simulink model "MODEL_SS_withSCC_Emily"  (R2024b)
settings: Solver=VariableStepAuto  StartTime=0.0  StopTime=40  RelTol=1e-3
PostLoadFcn:
  | Cconst = 0.15915494327;
  | Kp = [76; 141.7; 139.6; 114.2]*Cconst/60;
  | Tp = [14.4; 19.1; 9.39; 9.12];
  | Tg = 0.38*ones(4,1);
  | R = 3/60*ones(4,1);
  | Bagc = [0.416; 0.377; 0.378; 0.388]*60;
  | Kagc = [0.75; 0.25; 0.5; 0.5]*(-0.131);
  | Kdc = ones(4,1);
  | 
  | T = zeros(4,4);
  | T(1, 2) = 0.029;
  | T(1, 3) = 0.0143;
  | T(1, 4) = 0.0099;
  | T(2, 3) = 0.0205;
  | T(3, 4) = 0.0089;
  | T = T.*(60/Cconst);
  | T = T + T';
  | 
  | % State space of system with AGC
  | % x = [Pc Pg w Ptie]
  | % u = [Pl Pdc Pi+1 Pi+2 Pi+3]
  | % clear AMatrices BMatrices
  | AMatrices(4) = struct();
  | BMatrices(4) = struct();
  | for i = 1:4
  |     Amatrix = [
  |         0, 0, Kagc(i)*Bagc(i), Kagc(i)
  |         1/Tg(i), -1/Tg(i), -1/Tg(i)/R(i), 0
  |         0, Kp(i), -Tp(i), -Kp(i)
  |         0, 0, sum(T(i,:)), 0
  |     ];
  |     AMatrices(i).value = Amatrix;
  |     Bmatrix = [
  |         0,Kagc(i)*Kdc(i),0,0,0
  |         0,0,0,0,0
  |         -Kp(i),-Kp(i)*Kdc(i),0,0,0
  |         0,0,-T(i, mod(i,4)+1),-T(i, mod(i+1,4)+1),-T(i, mod(i+2,4)+1)
  |     ];
  |     BMatrices(i).value = Bmatrix;
  | end
  | 
  | % Safety Critical Controller system
  | % The input to this system also include the AGC inputs Pc
  | % x = [Pg w Ptie]1,2,3,4
  | % u = [Pc Pl Pdc]1,2,3,4
  | 
  | Ascc = [
  |     AMatrices(1).value(2:4, 2:4), ...
  |     [zeros(3,1), BMatrices(1).value(2:4,3), zeros(3,1)], ...
  |     [zeros(3,1), BMatrices(1).value(2:4,4), zeros(3,1)], ...
  |     [zeros(3,1), BMatrices(1).value(2:4,5), zeros(3,1)]
  | 
  |     [zeros(3,1), BMatrices(2).value(2:4,3), zeros(3,1)], ...
  |     AMatrices(2).value(2:4, 2:4), ...
  |     [zeros(3,1), BMatrices(2).value(2:4,4), zeros(3,1)], ...
  |     [zeros(3,1), BMatrices(2).value(2:4,5), zeros(3,1)]
  | 
  |     [zeros(3,1), BMatrices(3).value(2:4,3), zeros(3,1)], ...
  |     [zeros(3,1), BMatrices(3).value(2:4,4), zeros(3,1)], ...
  |     AMatrices(3).value(2:4, 2:4), ...
  |     [zeros(3,1), BMatrices(3).value(2:4,5), zeros(3,1)]
  | 
  |     [zeros(3,1), BMatrices(4).value(2:4,3), zeros(3,1)], ...
  |     [zeros(3,1), BMatrices(4).value(2:4,4), zeros(3,1)], ...
  |     [zeros(3,1), BMatrices(4).value(2:4,5), zeros(3,1)], ...
  |     AMatrices(4).value(2:4, 2:4)
  | ];
  | 
  | Bscc = [
  |     AMatrices(1).value(2:4, 1), ...
  |     BMatrices(1).value(2:4, 1:2), ...
  |     zeros(3, 9)
  | 
  |     zeros(3,3), ...
  |     AMatrices(2).value(2:4, 1), ...
  |     BMatrices(2).value(2:4, 1:2), ...
  |     zeros(3,6)
  | 
  |     zeros(3,6), ...
  |     AMatrices(3).value(2:4, 1), ...
  |     BMatrices(3).value(2:4, 1:2), ...
  |     zeros(3,3)
  | 
  |     zeros(3,9), ...
  |     AMatrices(4).value(2:4, 1), ...
  |     BMatrices(4).value(2:4, 1:2)
  | ];
  | 
  | C = zeros(4,12);
  | C(1,2) = 1; C(2,5) = 1; C(3,8) = 1; C(4,11) = 1; % extracting the frequencies
libraries: simulink x1
settings Model: Creator=amrmo  LastModifiedBy=amrmo

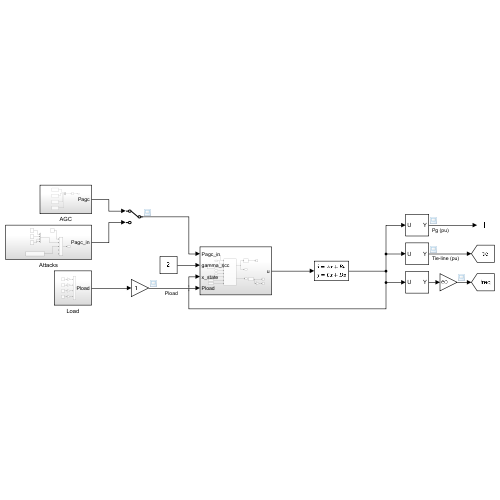
[thumbnail: Simulink's stored preview of the top-level diagram]
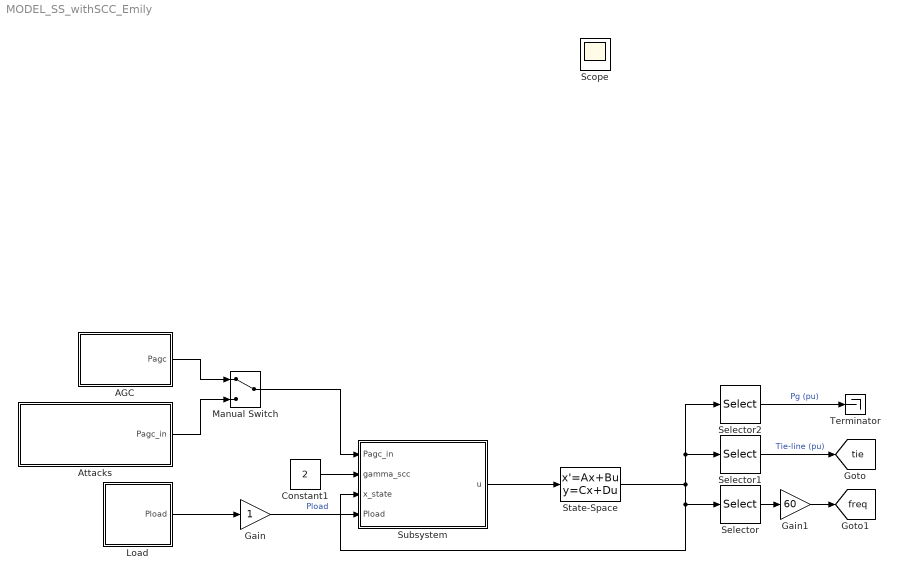
== system MODEL_SS_withSCC_Emily ==
  AGC : Subsystem
  Attacks : Subsystem
  Constant1 : Constant  Value=2
  Gain : Gain
  Gain1 : Gain  Gain=60
  Load : Subsystem
  Manual Switch : ManualSwitch
  Selector : Selector  InputPortWidth=12  IndexOptions=Index vector (dialog)  Indices=[2, 5, 8, 11]  OutputSizes=1
  Selector1 : Selector  InputPortWidth=12  IndexOptions=Index vector (dialog)  Indices=[3, 6, 9, 12]  OutputSizes=1
  Selector2 : Selector  InputPortWidth=12  IndexOptions=Index vector (dialog)  Indices=[1, 4, 7, 10]  OutputSizes=1
  State-Space : StateSpace  A=Ascc  B=Bscc  C=eye(size(Ascc,1))  D=zeros(size(Ascc,1), size(Bscc,2))  InitialCondition=0
  Subsystem : Subsystem
  Terminator : Terminator
  Scope : Scope
  tag scope: freq=global, tie=global
  wires:
  Selector/1 -> Gain1/1
  State-Space/1 -> Subsystem/3(x_state), Selector/1, Selector2/1, Selector1/1
  Selector1/1 -> [tie]  "Tie-line (pu)"
  Constant1/1 -> Subsystem/2(gamma_scc)
  Subsystem/1(u) -> State-Space/1
  Load/1(Pload) -> Gain/1
  Gain/1 -> Subsystem/4(Pload)  "Pload"
  AGC/1(Pagc) -> Manual Switch/1
  Manual Switch/1 -> Subsystem/1(Pagc_in)
  Selector2/1 -> Terminator/1  "Pg (pu)"
  Attacks/1(Pagc_in) -> Manual Switch/2
  Gain1/1 -> [freq]

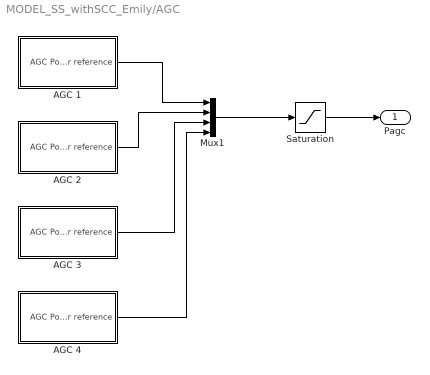
== system MODEL_SS_withSCC_Emily/AGC ==
  AGC 1 : Subsystem
  AGC 2 : Subsystem
  AGC 3 : Subsystem
  AGC 4 : Subsystem
  Mux1 : Mux
  Saturation : Saturate  UpperLimit=0.3  LowerLimit=-0.3
  Pagc : Outport
  wires:
  AGC 3/1(AGC Power reference) -> Mux1/3
  AGC 4/1(AGC Power reference) -> Mux1/4
  AGC 1/1(AGC Power reference) -> Mux1/1
  AGC 2/1(AGC Power reference) -> Mux1/2
  Mux1/1 -> Saturation/1
  Saturation/1 -> Pagc/1

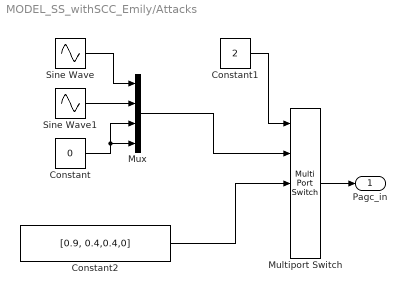
== system MODEL_SS_withSCC_Emily/Attacks ==
  Constant : Constant  Value=0
  Constant1 : Constant  Value=2
  Constant2 : Constant  Value=[0.9, 0.4,0.4,0]
  Multiport Switch : MultiPortSwitch  Inputs=4  SaturateOnIntegerOverflow=off  InputSameDT=off
  Mux : Mux
  Sine Wave : Sin  Amplitude=0.9  Frequency=3.497  SampleTime=0
  Sine Wave1 : Sin  Amplitude=0.7  Frequency=2.533  Phase=30*pi/180  SampleTime=0
  Pagc_in : Outport
  wires:
  Sine Wave/1 -> Mux/1
  Sine Wave1/1 -> Mux/2
  Constant/1 -> Mux/4, Mux/3
  Constant1/1 -> Multiport Switch/1
  Mux/1 -> Multiport Switch/2
  Constant2/1 -> Multiport Switch/3
  Multiport Switch/1 -> Pagc_in/1

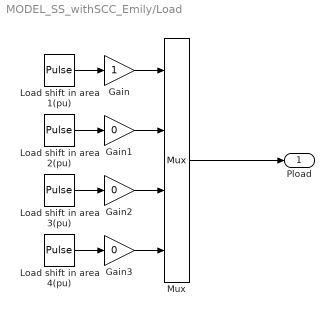
== system MODEL_SS_withSCC_Emily/Load ==
  Gain : Gain
  Gain1 : Gain  Gain=0
  Gain2 : Gain  Gain=0
  Gain3 : Gain  Gain=0
  Load shift in area 1(pu) : DiscretePulseGenerator  PulseType=Time based  Amplitude=0.1  Period=10  PulseWidth=25
  Load shift in area 2(pu) : DiscretePulseGenerator  PulseType=Time based  Amplitude=0.2  Period=2*pi/2.5  PulseWidth=40
  Load shift in area 3(pu) : DiscretePulseGenerator  PulseType=Time based  Amplitude=0  Period=10  PulseWidth=5
  Load shift in area 4(pu) : DiscretePulseGenerator  PulseType=Time based  Amplitude=0  Period=10  PulseWidth=5
  Mux : Mux
  Pload : Outport
  wires:
  Load shift in area 4(pu)/1 -> Gain3/1
  Load shift in area 2(pu)/1 -> Gain1/1
  Load shift in area 3(pu)/1 -> Gain2/1
  Load shift in area 1(pu)/1 -> Gain/1
  Mux/1 -> Pload/1
  Gain/1 -> Mux/1
  Gain1/1 -> Mux/2
  Gain2/1 -> Mux/3
  Gain3/1 -> Mux/4

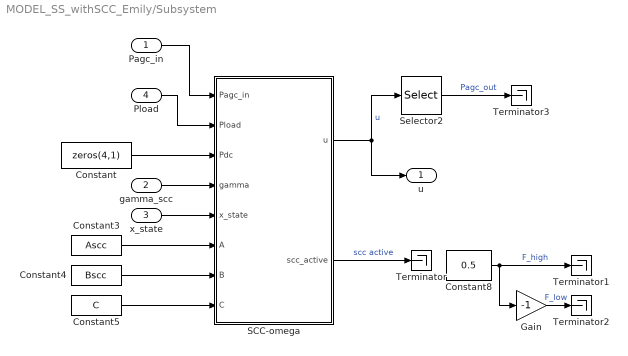
== system MODEL_SS_withSCC_Emily/Subsystem ==
  Pagc_in : Inport
  gamma_scc : Inport  Port=2
  x_state : Inport  Port=3
  Pload : Inport  Port=4
  Constant : Constant  Value=zeros(4,1)
  Constant3 : Constant  Value=Ascc
  Constant4 : Constant  Value=Bscc
  Constant5 : Constant  Value=C
  Constant8 : Constant  Value=0.5
  Gain : Gain  Gain=-1
  SCC-omega : MATLAB Function  TreatAsAtomicUnit=on
  Selector2 : Selector  InputPortWidth=12  IndexOptions=Index vector (dialog)  Indices=[1 4 7 10]  OutputSizes=1
  Terminator{,1..3} (4 alike) : Terminator
  u : Outport
  wires:
  Pload/1 -> SCC-omega/2(Pload)
  Constant5/1 -> SCC-omega/8(C)
  Constant3/1 -> SCC-omega/6(A)
  Constant/1 -> SCC-omega/3(Pdc)
  SCC-omega/1(u) -> u/1, Selector2/1  "u"
  Selector2/1 -> Terminator3/1  "Pagc_out"
  Constant4/1 -> SCC-omega/7(B)
  x_state/1 -> SCC-omega/5(x_state)
  gamma_scc/1 -> SCC-omega/4(gamma)
  Pagc_in/1 -> SCC-omega/1(Pagc_in)
  SCC-omega/2(scc_active) -> Terminator/1  "scc active"
  Constant8/1 -> Terminator1/1, Gain/1  "F_high"
  Gain/1 -> Terminator2/1  "F_low"

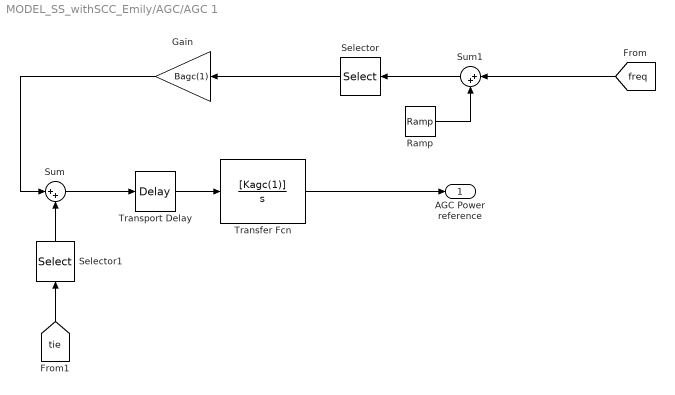
== system MODEL_SS_withSCC_Emily/AGC/AGC 1 ==
  Gain : Gain  Gain=Bagc(1)
  Ramp : simulink/Sources/Ramp  slope=0.02*0  start=0  InitialOutput=0
  Selector : Selector  InputPortWidth=4  IndexOptions=Index vector (dialog)  Indices=[1]  OutputSizes=1
  Selector1 : Selector  InputPortWidth=4  IndexOptions=Index vector (dialog)  Indices=[1]  OutputSizes=1
  Sum : Sum  Inputs=|++
  Sum1 : Sum  Inputs=|++
  Transfer Fcn : TransferFcn  Numerator=[Kagc(1)]  Denominator=[1 0]
  Transport Delay : TransportDelay  DelayTime=0
  AGC Power reference : Outport
  wires:
  Sum/1 -> Transport Delay/1
  Gain/1 -> Sum/1
  Selector/1 -> Gain/1
  Selector1/1 -> Sum/2
  [tie] -> Selector1/1
  Sum1/1 -> Selector/1
  Ramp/1 -> Sum1/2
  [freq] -> Sum1/1
  Transport Delay/1 -> Transfer Fcn/1
  Transfer Fcn/1 -> AGC Power reference/1

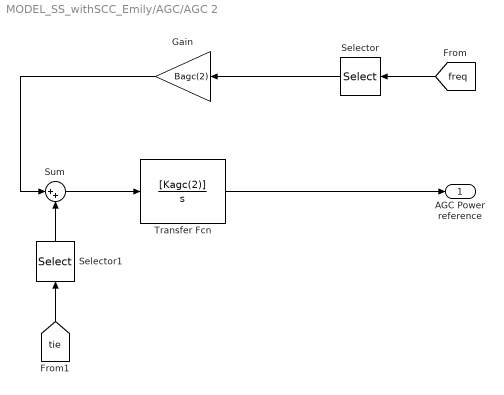
== system MODEL_SS_withSCC_Emily/AGC/AGC 2 ==
  Gain : Gain  Gain=Bagc(2)
  Selector : Selector  InputPortWidth=4  IndexOptions=Index vector (dialog)  Indices=[2]  OutputSizes=1
  Selector1 : Selector  InputPortWidth=4  IndexOptions=Index vector (dialog)  Indices=[2]  OutputSizes=1
  Sum : Sum  Inputs=|++
  Transfer Fcn : TransferFcn  Numerator=[Kagc(2)]  Denominator=[1 0]
  AGC Power reference : Outport
  wires:
  Sum/1 -> Transfer Fcn/1
  Gain/1 -> Sum/1
  Selector/1 -> Gain/1
  Selector1/1 -> Sum/2
  [freq] -> Selector/1
  [tie] -> Selector1/1
  Transfer Fcn/1 -> AGC Power reference/1

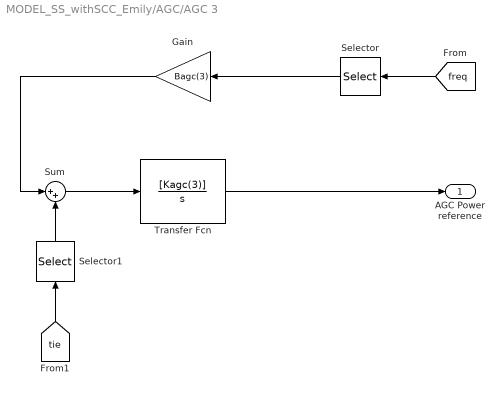
== system MODEL_SS_withSCC_Emily/AGC/AGC 3 ==
  Gain : Gain  Gain=Bagc(3)
  Selector : Selector  InputPortWidth=4  IndexOptions=Index vector (dialog)  Indices=[3]  OutputSizes=1
  Selector1 : Selector  InputPortWidth=4  IndexOptions=Index vector (dialog)  Indices=[3]  OutputSizes=1
  Sum : Sum  Inputs=|++
  Transfer Fcn : TransferFcn  Numerator=[Kagc(3)]  Denominator=[1 0]
  AGC Power reference : Outport
  wires:
  Transfer Fcn/1 -> AGC Power reference/1
  Sum/1 -> Transfer Fcn/1
  Gain/1 -> Sum/1
  Selector/1 -> Gain/1
  Selector1/1 -> Sum/2
  [freq] -> Selector/1
  [tie] -> Selector1/1

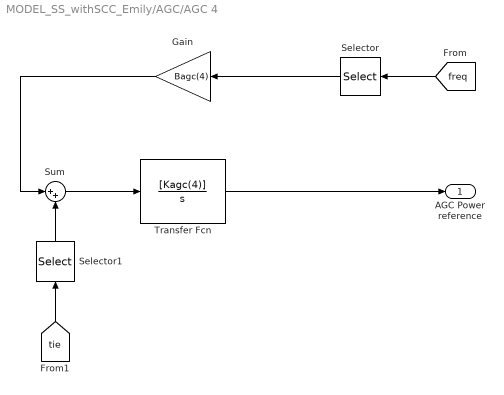
== system MODEL_SS_withSCC_Emily/AGC/AGC 4 ==
  Gain : Gain  Gain=Bagc(4)
  Selector : Selector  InputPortWidth=4  IndexOptions=Index vector (dialog)  Indices=[4]  OutputSizes=1
  Selector1 : Selector  InputPortWidth=4  IndexOptions=Index vector (dialog)  Indices=[4]  OutputSizes=1
  Sum : Sum  Inputs=|++
  Transfer Fcn : TransferFcn  Numerator=[Kagc(4)]  Denominator=[1 0]
  AGC Power reference : Outport
  wires:
  Transfer Fcn/1 -> AGC Power reference/1
  Sum/1 -> Transfer Fcn/1
  Gain/1 -> Sum/1
  Selector/1 -> Gain/1
  Selector1/1 -> Sum/2
  [freq] -> Selector/1
  [tie] -> Selector1/1

== matlab function MODEL_SS_withSCC_Emily/Subsystem/SCC-omega ==
  data: Pagc_in input; u output; Pload input; Pdc input; gamma input; scc_active output; x_state input; A input; B input; C input
function [u, scc_active] = fcn(Pagc_in, Pload, Pdc, gamma , x_state, ...
    A, B, C)
    %{
        INPUTS: 
        - Pagc_in: float(4,1): is the agc control signal (pu) to each of areas 1, 2, 3, 4
        - Pload: float(4,1): is the load change (pu) in areas 1, 2, 3, 4
        - Pdc: float(4,1): is the dc power injection (pu) to areas 1, 2, 3, 4
        - x_state: float(12,1): is the state of the system [Pg (pu), frequency (pu), Ptie
        (pu)]1,2,3,4
        
        - alpha_scc: float(1,1): is the alpha parameter of the safety-critical controller.
        alpha_scc = 0 deactivates the safety critical controller.
        Lower alpha_scc makes the safety critical controller less relaxed.
        
        OUTPUTS:
        - u: float(12,1): is the input to the system consisting of [Pagc (pu), Pload (pu), 
        Pds (pu)]1,2,3,4
        - scc_active \in {0,1} is a boolean for whether the safety critical controller
        was activated or not.
        
    %}
    coder.extrinsic('safety_critical_controller');
    u = zeros(12,1);
    scc_active = 0;
    [u, scc_active] = safety_critical_controller(Pagc_in, Pload, Pdc, gamma , x_state, ...
    A, B, C);
end
